simulink model "lqr_lqe"  (R2024b)
settings: Solver=ode4  StartTime=0.0  StopTime=T  FixedStep=Ts  RelTol=1e-3
values from neighbouring files (symbols this model uses):
  D = [0 0]'    [IP_MACRO.m]
  K = lqr(A, B, Qr, Rr)    [IP_MACRO.m]
  L = lqe(A, G, C, Qe, Re)    [IP_MACRO.m]
  x0 = [0.1 1 0.2 0 0]'    [IP_MACRO.m]
undefined symbols (not defined in the file or in its folder): A, B, C
settings Model: Creator=leita  LastModifiedBy=leita
settings DataIOCC: ReturnWorkspaceOutputs=off

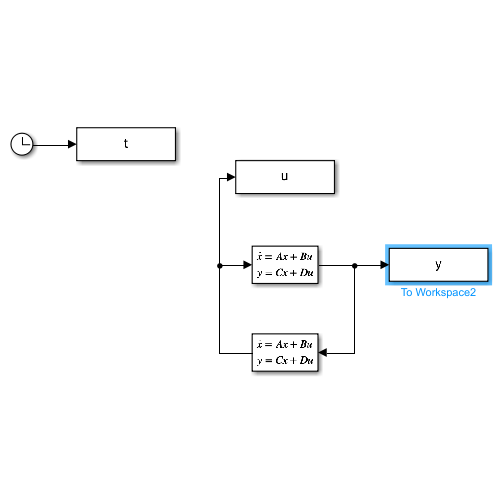
[thumbnail: Simulink's stored preview of the top-level diagram]
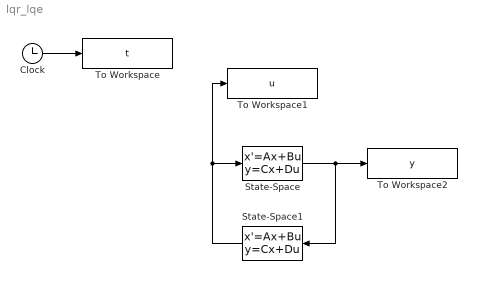
== system lqr_lqe ==
  Clock : Clock
  State-Space : StateSpace  A=A  B=B  C=C  D=D  InitialCondition=x0
  State-Space1 : StateSpace  A=A-B*K-L*C  B=L  C=-K  D=[0,0]  InitialCondition=0
  To Workspace : ToWorkspace  VariableName=t  SaveFormat=Timeseries  SampleTime=-1
  To Workspace1 : ToWorkspace  VariableName=u  SaveFormat=Timeseries  SampleTime=-1
  To Workspace2 : ToWorkspace  VariableName=y  SaveFormat=Timeseries  SampleTime=-1
  wires:
  Clock/1 -> To Workspace/1
  State-Space1/1 -> To Workspace1/1, State-Space/1
  State-Space/1 -> State-Space1/1, To Workspace2/1
